simulink model "ConditionTransitionAction"  (R2020b)
settings: Solver=VariableStepAuto  StartTime=0.0  StopTime=10.0  RelTol=1e-3
settings Model: Creator=apple  LastModifiedBy=apple

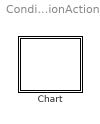
== system ConditionTransitionAction ==
  Chart : Stateflow chart  TreatAsAtomicUnit=on

== stateflow chart ConditionTransitionAction/Chart ==
  state A
    en:fprintf("Entry A");
    du:fprintf("During A");
    ex:fprintf("Exit A");
  state B
    en:fprintf("Entry B");
    du:fprintf("During B");
    ex:fprintf("Exit B");
  (default) -> A : {x= 0;}
  A -> B : E_one[x > -1]{fprintf("Condition Action");}/{fprintf("Transition Action");}
  B -> A : E_two
  data: x local
  events: E_two local FUNCTION_CALL_EVENT; E_one local FUNCTION_CALL_EVENT
